simulink model "TestSolidStateTransformer"  (R2025b)
settings: Solver=VariableStepAuto  StartTime=0.0  StopTime=0.5  FixedStep=50e-6  RelTol=1e-3
model workspace (MAT data in the model file):
  sst : object (value not decoded)
  ups : sampleTime (value not decoded)
symbols that are objects in the model workspace (value not decoded): ups
undefined symbols (not defined in the file): DiscIntNeverNeededParam, ee_sli_rtmsupport, gcbh, Ts
libraries: fl_lib x23, nesl_utility x20, datacenter_lib x12, ee_lib x9, simulink x8, eeGeneralControl x6, eeTransforms x4, slpidlib x3, eeSinusoidalMeasurementV2 x2, simulink_extras x1
(part 2 of 2)

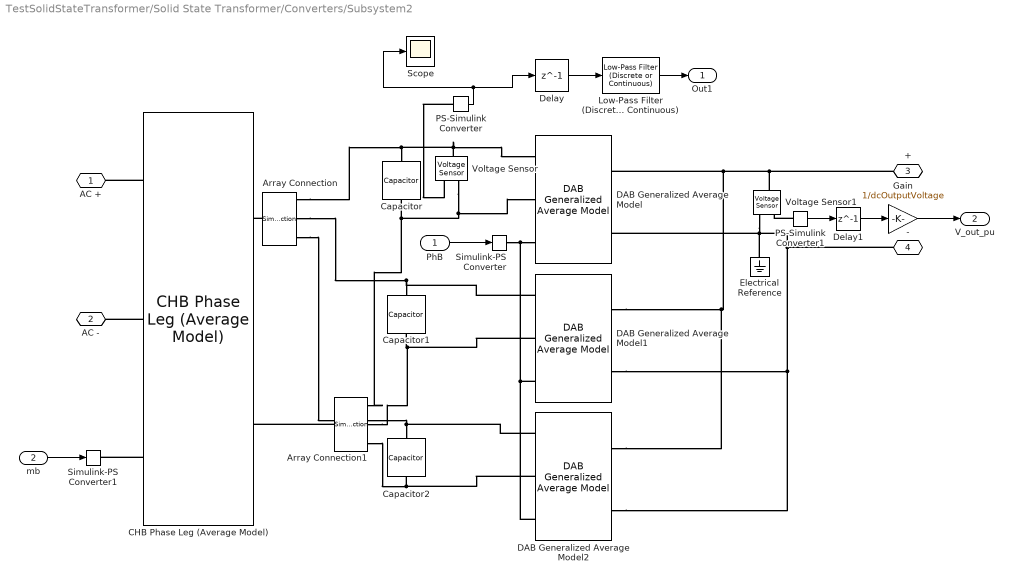
== system TestSolidStateTransformer/Solid State Transformer/Converters/Subsystem2 ==
  PhB : Inport
  mb : Inport  Port=2
  Array Connection : SimscapeArrayConnection  NumScalarElements=3
  Array Connection1 : SimscapeArrayConnection  NumScalarElements=3
  CHB Phase Leg (Average Model) : datacenter_lib/CHB Phase Leg (Average Model)  NumModules=3  OnResistance=1e-3 Ohm  InitialDCVoltage=4400 V  GridVoltage=13800 V  TotalDCVoltage=13200 V
      settings: InternalSimscapePortConfiguration="{\"Bottom\":[],\"Left\":[{\"id\":\"ACPositive\",\"label\":\"AC+\",\"type\":\"foundation.electrical.electrical\"},{\"id\":\"ACNegative\",\"label\":\"AC-\",\"type\":\"foundation.electrical.electrical\"},{\"id\":\"m\",\"label\":\"m\",\"type\":\"input\"}],\"Right\":[{\"id\":\"DCPositive\",\"label\":\"DC+\",\"type\":\"foundation.electrical.electrical\"},{\"id\":\"DCNegative\",\"label\":\"DC-\",\"type\":\"foundation.electrical.electrical\"}],\"Top\":[]}"
  Capacitor : fl_lib/Electrical/Electrical Elements/Capacitor  c=0.005 F  r=1e-6 Ohm  g=0 1/Ohm  i_specify=off  i_priority=None  i=0 A  i_nominal_specify=off  i_nominal_value=1  i_nominal_unit=A  v_specify=off  v_priority=None  v=0 V  v_nominal_specify=off  v_nominal_value=1  v_nominal_unit=V  vc_specify=on  vc_priority=None  vc=4400 V  vc_nominal_specify=off  vc_nominal_value=1  vc_nominal_unit=V
  Capacitor1 : fl_lib/Electrical/Electrical Elements/Capacitor  c=0.005 F  r=1e-6 Ohm  g=0 1/Ohm  i_specify=off  i_priority=None  i=0 A  i_nominal_specify=off  i_nominal_value=1  i_nominal_unit=A  v_specify=off  v_priority=None  v=0 V  v_nominal_specify=off  v_nominal_value=1  v_nominal_unit=V  vc_specify=on  vc_priority=None  vc=4400 V  vc_nominal_specify=off  vc_nominal_value=1  vc_nominal_unit=V
  Capacitor2 : fl_lib/Electrical/Electrical Elements/Capacitor  c=0.005 F  r=1e-6 Ohm  g=0 1/Ohm  i_specify=off  i_priority=None  i=0 A  i_nominal_specify=off  i_nominal_value=1  i_nominal_unit=A  v_specify=off  v_priority=None  v=0 V  v_nominal_specify=off  v_nominal_value=1  v_nominal_unit=V  vc_specify=on  vc_priority=None  vc=4400 V  vc_nominal_specify=off  vc_nominal_value=1  vc_nominal_unit=V
  DAB Generalized Average Model : datacenter_lib/DAB Generalized Average Model  N=5.5  L1=3.4e-05 H  L2=1.12e-06 H  Rt=0.005 Ohm  Co=0.001 F  fs=20000 Hz  vo0_init=800 V  it1R_init=0 A  it1I_init=0 A  include_esr=false  Rc=0.25 Ohm  i_in_specify=on  i_in_priority=None  i_in=0 A  i_in_nominal_specify=off  i_in_nominal_value=1  i_in_nominal_unit=A  i_out_specify=on  i_out_priority=None  i_out=0 A  i_out_nominal_specify=off  i_out_nominal_value=1  i_out_nominal_unit=A  v_in_specify=on  v_in_priority=None  v_in=0 V  v_in_nominal_specify=off  v_in_nominal_value=1  v_in_nominal_unit=V  v_out_specify=on  v_out_priority=None  v_out=0 V  v_out_nominal_specify=off  v_out_nominal_value=1  v_out_nominal_unit=V
      settings: InternalSimscapePortConfiguration="{\"Bottom\":[],\"Left\":[{\"id\":\"p_in\",\"label\":\"V+\",\"type\":\"foundation.electrical.electrical\"},{\"id\":\"n_in\",\"label\":\"V-\",\"type\":\"foundation.electrical.electrical\"},{\"id\":\"d\",\"label\":\"d\",\"type\":\"input\"}],\"Right\":[{\"id\":\"p_out\",\"label\":\"Vo+\",\"type\":\"foundation.electrical.electrical\"},{\"id\":\"n_out\",\"label\":\"Vo-\",\"type\":\"foundation.electrical.electrical\"}],\"Top\":[]}"
  DAB Generalized Average Model1 : datacenter_lib/DAB Generalized Average Model  N=5.5  L1=3.4e-05 H  L2=1.12e-06 H  Rt=0.005 Ohm  Co=0.001 F  fs=20000 Hz  vo0_init=800 V  it1R_init=0 A  it1I_init=0 A  include_esr=false  Rc=0.25 Ohm  i_in_specify=on  i_in_priority=None  i_in=0 A  i_in_nominal_specify=off  i_in_nominal_value=1  i_in_nominal_unit=A  i_out_specify=on  i_out_priority=None  i_out=0 A  i_out_nominal_specify=off  i_out_nominal_value=1  i_out_nominal_unit=A  v_in_specify=on  v_in_priority=None  v_in=0 V  v_in_nominal_specify=off  v_in_nominal_value=1  v_in_nominal_unit=V  v_out_specify=on  v_out_priority=None  v_out=0 V  v_out_nominal_specify=off  v_out_nominal_value=1  v_out_nominal_unit=V
      settings: InternalSimscapePortConfiguration="{\"Bottom\":[],\"Left\":[{\"id\":\"p_in\",\"label\":\"V+\",\"type\":\"foundation.electrical.electrical\"},{\"id\":\"n_in\",\"label\":\"V-\",\"type\":\"foundation.electrical.electrical\"},{\"id\":\"d\",\"label\":\"d\",\"type\":\"input\"}],\"Right\":[{\"id\":\"p_out\",\"label\":\"Vo+\",\"type\":\"foundation.electrical.electrical\"},{\"id\":\"n_out\",\"label\":\"Vo-\",\"type\":\"foundation.electrical.electrical\"}],\"Top\":[]}"
  DAB Generalized Average Model2 : datacenter_lib/DAB Generalized Average Model  N=5.5  L1=3.4e-05 H  L2=1.12e-06 H  Rt=0.005 Ohm  Co=0.001 F  fs=20000 Hz  vo0_init=800 V  it1R_init=0 A  it1I_init=0 A  include_esr=false  Rc=0.25 Ohm  i_in_specify=on  i_in_priority=None  i_in=0 A  i_in_nominal_specify=off  i_in_nominal_value=1  i_in_nominal_unit=A  i_out_specify=on  i_out_priority=None  i_out=0 A  i_out_nominal_specify=off  i_out_nominal_value=1  i_out_nominal_unit=A  v_in_specify=on  v_in_priority=None  v_in=0 V  v_in_nominal_specify=off  v_in_nominal_value=1  v_in_nominal_unit=V  v_out_specify=on  v_out_priority=None  v_out=0 V  v_out_nominal_specify=off  v_out_nominal_value=1  v_out_nominal_unit=V
      settings: InternalSimscapePortConfiguration="{\"Bottom\":[],\"Left\":[{\"id\":\"p_in\",\"label\":\"V+\",\"type\":\"foundation.electrical.electrical\"},{\"id\":\"n_in\",\"label\":\"V-\",\"type\":\"foundation.electrical.electrical\"},{\"id\":\"d\",\"label\":\"d\",\"type\":\"input\"}],\"Right\":[{\"id\":\"p_out\",\"label\":\"Vo+\",\"type\":\"foundation.electrical.electrical\"},{\"id\":\"n_out\",\"label\":\"Vo-\",\"type\":\"foundation.electrical.electrical\"}],\"Top\":[]}"
  Delay : Delay  DelayLength=1
  Delay1 : Delay  DelayLength=1  InitialCondition=1
  Electrical Reference : fl_lib/Electrical/Electrical Elements/Electrical Reference
  Gain : Gain  Gain=1/dcOutputVoltage
  Low-Pass Filter (Discrete or Continuous) : eeGeneralControl/Low-Pass Filter (Discrete or Continuous)  K=1  T=0.005  B=inf  A=-inf  init_option=Inherited from block input  x0=0  Ts=-1
  PS-Simulink Converter : nesl_utility/PS-Simulink Converter  PhysicalDomain=network_engine_domain  SubClassName=ps_output  LeftPortType=input  RightPortType=output  PseudoPeriodic=off  Frequencies=[]  VectorFormat=inherit  Unit=inherit  AffineConversion=off
  PS-Simulink Converter1 : nesl_utility/PS-Simulink Converter  PhysicalDomain=network_engine_domain  SubClassName=ps_output  LeftPortType=input  RightPortType=output  PseudoPeriodic=off  Frequencies=[]  VectorFormat=inherit  Unit=inherit  AffineConversion=off
  Scope : Scope
      settings: ActiveDisplayYMinimum=-1  ActiveDisplayYMaximum=1
  Simulink-PS Converter : nesl_utility/Simulink-PS Converter  PhysicalDomain=network_engine_domain  SubClassName=ps_input  LeftPortType=input  RightPortType=output  PseudoPeriodic=off  Frequencies=[]  NoiseDistribution=none  NoiseParameters=[]  Unit=1  AffineConversion=off  FilteringAndDerivatives=provide  SimscapeFilterOrder=1  InputFilterTimeConstant=0.001  UdotUserProvided=0
  Simulink-PS Converter1 : nesl_utility/Simulink-PS Converter  PhysicalDomain=network_engine_domain  SubClassName=ps_input  LeftPortType=input  RightPortType=output  PseudoPeriodic=off  Frequencies=[]  NoiseDistribution=none  NoiseParameters=[]  Unit=1  AffineConversion=off  FilteringAndDerivatives=provide  SimscapeFilterOrder=1  InputFilterTimeConstant=0.001  UdotUserProvided=0
  Voltage Sensor : fl_lib/Electrical/Electrical Sensors/Voltage Sensor
  Voltage Sensor1 : fl_lib/Electrical/Electrical Sensors/Voltage Sensor
  AC + : PMIOPort  Side=Left
  AC - : PMIOPort  Port=2  Side=Left
  + : PMIOPort  Port=3  Side=Right
  - : PMIOPort  Port=4  Side=Right
  Out1 : Outport
  V_out_pu : Outport  Port=2
  wires:
  mb/1 -> Simulink-PS Converter1/1
  Gain/1 -> V_out_pu/1
  PhB/1 -> Simulink-PS Converter/1
  Delay1/1 -> Gain/1
  PS-Simulink Converter1/1 -> Delay1/1
  Low-Pass Filter (Discrete or Continuous)/1 -> Out1/1
  Delay/1 -> Low-Pass Filter (Discrete or Continuous)/1
  PS-Simulink Converter/1 -> Scope/1, Delay/1
  connections:
  CHB Phase Leg (Average Model)/LConn3 -- Simulink-PS Converter1/RConn1
  Array Connection1/RConn1 -- CHB Phase Leg (Average Model)/RConn2
  Array Connection/RConn1 -- CHB Phase Leg (Average Model)/RConn1
  DAB Generalized Average Model/LConn3 -- DAB Generalized Average Model1/LConn3 -- DAB Generalized Average Model2/LConn3 -- Simulink-PS Converter/RConn1
  PS-Simulink Converter1/LConn1 -- Voltage Sensor1/RConn1
  DAB Generalized Average Model1/RConn2 -- DAB Generalized Average Model2/RConn2 -- DAB Generalized Average Model/RConn2 -- Voltage Sensor1/RConn2 -- Electrical Reference/LConn1 -- -/RConn1
  DAB Generalized Average Model/RConn1 -- DAB Generalized Average Model1/RConn1 -- DAB Generalized Average Model2/RConn1 -- Voltage Sensor1/LConn1 -- +/RConn1
  Capacitor/RConn1 -- DAB Generalized Average Model/LConn2 -- Voltage Sensor/RConn2 -- Array Connection1/LConn1
  CHB Phase Leg (Average Model)/LConn2 -- AC -/RConn1
  Array Connection/LConn3 -- DAB Generalized Average Model2/LConn1 -- Capacitor2/LConn1
  Array Connection1/LConn3 -- Capacitor2/RConn1 -- DAB Generalized Average Model2/LConn2
  CHB Phase Leg (Average Model)/LConn1 -- AC +/RConn1
  Array Connection/LConn1 -- DAB Generalized Average Model/LConn1 -- Voltage Sensor/LConn1 -- Capacitor/LConn1
  Array Connection1/LConn2 -- DAB Generalized Average Model1/LConn2 -- Capacitor1/RConn1
  Array Connection/LConn2 -- Capacitor1/LConn1 -- DAB Generalized Average Model1/LConn1
  PS-Simulink Converter/LConn1 -- Voltage Sensor/RConn1

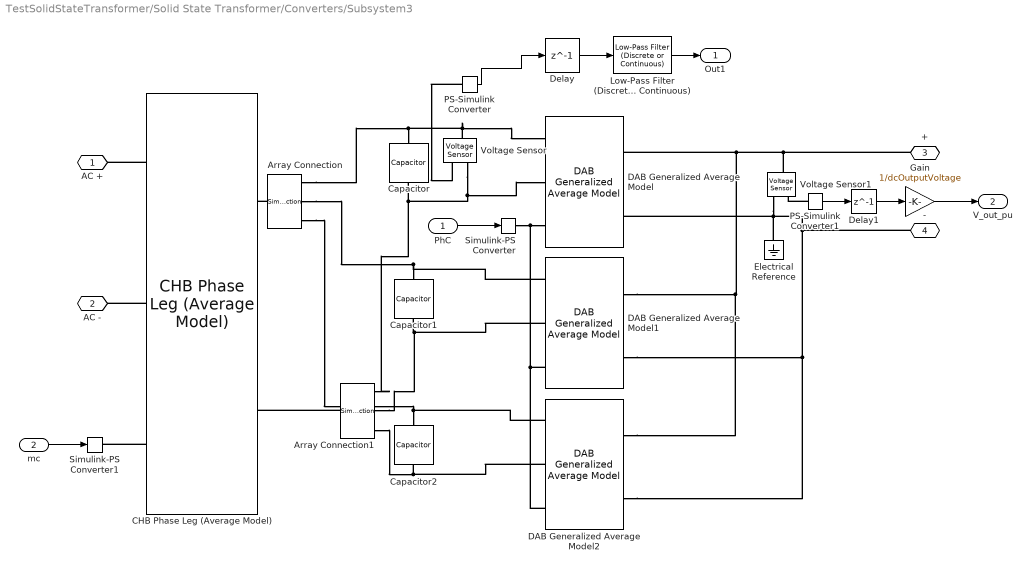
== system TestSolidStateTransformer/Solid State Transformer/Converters/Subsystem3 ==
  PhC : Inport
  mc : Inport  Port=2
  Array Connection : SimscapeArrayConnection  NumScalarElements=3
  Array Connection1 : SimscapeArrayConnection  NumScalarElements=3
  CHB Phase Leg (Average Model) : datacenter_lib/CHB Phase Leg (Average Model)  NumModules=3  OnResistance=1e-3 Ohm  InitialDCVoltage=4400 V  GridVoltage=13800 V  TotalDCVoltage=13200 V
      settings: InternalSimscapePortConfiguration="{\"Bottom\":[],\"Left\":[{\"id\":\"ACPositive\",\"label\":\"AC+\",\"type\":\"foundation.electrical.electrical\"},{\"id\":\"ACNegative\",\"label\":\"AC-\",\"type\":\"foundation.electrical.electrical\"},{\"id\":\"m\",\"label\":\"m\",\"type\":\"input\"}],\"Right\":[{\"id\":\"DCPositive\",\"label\":\"DC+\",\"type\":\"foundation.electrical.electrical\"},{\"id\":\"DCNegative\",\"label\":\"DC-\",\"type\":\"foundation.electrical.electrical\"}],\"Top\":[]}"
  Capacitor : fl_lib/Electrical/Electrical Elements/Capacitor  c=0.005 F  r=1e-6 Ohm  g=0 1/Ohm  i_specify=off  i_priority=None  i=0 A  i_nominal_specify=off  i_nominal_value=1  i_nominal_unit=A  v_specify=off  v_priority=None  v=0 V  v_nominal_specify=off  v_nominal_value=1  v_nominal_unit=V  vc_specify=on  vc_priority=None  vc=4400 V  vc_nominal_specify=off  vc_nominal_value=1  vc_nominal_unit=V
  Capacitor1 : fl_lib/Electrical/Electrical Elements/Capacitor  c=0.005 F  r=1e-6 Ohm  g=0 1/Ohm  i_specify=off  i_priority=None  i=0 A  i_nominal_specify=off  i_nominal_value=1  i_nominal_unit=A  v_specify=off  v_priority=None  v=0 V  v_nominal_specify=off  v_nominal_value=1  v_nominal_unit=V  vc_specify=on  vc_priority=None  vc=4400 V  vc_nominal_specify=off  vc_nominal_value=1  vc_nominal_unit=V
  Capacitor2 : fl_lib/Electrical/Electrical Elements/Capacitor  c=0.005 F  r=1e-6 Ohm  g=0 1/Ohm  i_specify=off  i_priority=None  i=0 A  i_nominal_specify=off  i_nominal_value=1  i_nominal_unit=A  v_specify=off  v_priority=None  v=0 V  v_nominal_specify=off  v_nominal_value=1  v_nominal_unit=V  vc_specify=on  vc_priority=None  vc=4400 V  vc_nominal_specify=off  vc_nominal_value=1  vc_nominal_unit=V
  DAB Generalized Average Model : datacenter_lib/DAB Generalized Average Model  N=5.5  L1=3.4e-05 H  L2=1.12e-06 H  Rt=0.005 Ohm  Co=0.001 F  fs=20000 Hz  vo0_init=800 V  it1R_init=0 A  it1I_init=0 A  include_esr=false  Rc=0.25 Ohm  i_in_specify=on  i_in_priority=None  i_in=0 A  i_in_nominal_specify=off  i_in_nominal_value=1  i_in_nominal_unit=A  i_out_specify=on  i_out_priority=None  i_out=0 A  i_out_nominal_specify=off  i_out_nominal_value=1  i_out_nominal_unit=A  v_in_specify=on  v_in_priority=None  v_in=0 V  v_in_nominal_specify=off  v_in_nominal_value=1  v_in_nominal_unit=V  v_out_specify=on  v_out_priority=None  v_out=0 V  v_out_nominal_specify=off  v_out_nominal_value=1  v_out_nominal_unit=V
      settings: InternalSimscapePortConfiguration="{\"Bottom\":[],\"Left\":[{\"id\":\"p_in\",\"label\":\"V+\",\"type\":\"foundation.electrical.electrical\"},{\"id\":\"n_in\",\"label\":\"V-\",\"type\":\"foundation.electrical.electrical\"},{\"id\":\"d\",\"label\":\"d\",\"type\":\"input\"}],\"Right\":[{\"id\":\"p_out\",\"label\":\"Vo+\",\"type\":\"foundation.electrical.electrical\"},{\"id\":\"n_out\",\"label\":\"Vo-\",\"type\":\"foundation.electrical.electrical\"}],\"Top\":[]}"
  DAB Generalized Average Model1 : datacenter_lib/DAB Generalized Average Model  N=5.5  L1=3.4e-05 H  L2=1.12e-06 H  Rt=0.005 Ohm  Co=0.001 F  fs=20000 Hz  vo0_init=800 V  it1R_init=0 A  it1I_init=0 A  include_esr=false  Rc=0.25 Ohm  i_in_specify=on  i_in_priority=None  i_in=0 A  i_in_nominal_specify=off  i_in_nominal_value=1  i_in_nominal_unit=A  i_out_specify=on  i_out_priority=None  i_out=0 A  i_out_nominal_specify=off  i_out_nominal_value=1  i_out_nominal_unit=A  v_in_specify=on  v_in_priority=None  v_in=0 V  v_in_nominal_specify=off  v_in_nominal_value=1  v_in_nominal_unit=V  v_out_specify=on  v_out_priority=None  v_out=0 V  v_out_nominal_specify=off  v_out_nominal_value=1  v_out_nominal_unit=V
      settings: InternalSimscapePortConfiguration="{\"Bottom\":[],\"Left\":[{\"id\":\"p_in\",\"label\":\"V+\",\"type\":\"foundation.electrical.electrical\"},{\"id\":\"n_in\",\"label\":\"V-\",\"type\":\"foundation.electrical.electrical\"},{\"id\":\"d\",\"label\":\"d\",\"type\":\"input\"}],\"Right\":[{\"id\":\"p_out\",\"label\":\"Vo+\",\"type\":\"foundation.electrical.electrical\"},{\"id\":\"n_out\",\"label\":\"Vo-\",\"type\":\"foundation.electrical.electrical\"}],\"Top\":[]}"
  DAB Generalized Average Model2 : datacenter_lib/DAB Generalized Average Model  N=5.5  L1=3.4e-05 H  L2=1.12e-06 H  Rt=0.005 Ohm  Co=0.001 F  fs=20000 Hz  vo0_init=800 V  it1R_init=0 A  it1I_init=0 A  include_esr=false  Rc=0.25 Ohm  i_in_specify=on  i_in_priority=None  i_in=0 A  i_in_nominal_specify=off  i_in_nominal_value=1  i_in_nominal_unit=A  i_out_specify=on  i_out_priority=None  i_out=0 A  i_out_nominal_specify=off  i_out_nominal_value=1  i_out_nominal_unit=A  v_in_specify=on  v_in_priority=None  v_in=0 V  v_in_nominal_specify=off  v_in_nominal_value=1  v_in_nominal_unit=V  v_out_specify=on  v_out_priority=None  v_out=0 V  v_out_nominal_specify=off  v_out_nominal_value=1  v_out_nominal_unit=V
      settings: InternalSimscapePortConfiguration="{\"Bottom\":[],\"Left\":[{\"id\":\"p_in\",\"label\":\"V+\",\"type\":\"foundation.electrical.electrical\"},{\"id\":\"n_in\",\"label\":\"V-\",\"type\":\"foundation.electrical.electrical\"},{\"id\":\"d\",\"label\":\"d\",\"type\":\"input\"}],\"Right\":[{\"id\":\"p_out\",\"label\":\"Vo+\",\"type\":\"foundation.electrical.electrical\"},{\"id\":\"n_out\",\"label\":\"Vo-\",\"type\":\"foundation.electrical.electrical\"}],\"Top\":[]}"
  Delay : Delay  DelayLength=1
  Delay1 : Delay  DelayLength=1  InitialCondition=1
  Electrical Reference : fl_lib/Electrical/Electrical Elements/Electrical Reference
  Gain : Gain  Gain=1/dcOutputVoltage
  Low-Pass Filter (Discrete or Continuous) : eeGeneralControl/Low-Pass Filter (Discrete or Continuous)  K=1  T=0.005  B=inf  A=-inf  init_option=Inherited from block input  x0=0  Ts=-1
  PS-Simulink Converter : nesl_utility/PS-Simulink Converter  PhysicalDomain=network_engine_domain  SubClassName=ps_output  LeftPortType=input  RightPortType=output  PseudoPeriodic=off  Frequencies=[]  VectorFormat=inherit  Unit=inherit  AffineConversion=off
  PS-Simulink Converter1 : nesl_utility/PS-Simulink Converter  PhysicalDomain=network_engine_domain  SubClassName=ps_output  LeftPortType=input  RightPortType=output  PseudoPeriodic=off  Frequencies=[]  VectorFormat=inherit  Unit=inherit  AffineConversion=off
  Simulink-PS Converter : nesl_utility/Simulink-PS Converter  PhysicalDomain=network_engine_domain  SubClassName=ps_input  LeftPortType=input  RightPortType=output  PseudoPeriodic=off  Frequencies=[]  NoiseDistribution=none  NoiseParameters=[]  Unit=1  AffineConversion=off  FilteringAndDerivatives=provide  SimscapeFilterOrder=1  InputFilterTimeConstant=0.001  UdotUserProvided=0
  Simulink-PS Converter1 : nesl_utility/Simulink-PS Converter  PhysicalDomain=network_engine_domain  SubClassName=ps_input  LeftPortType=input  RightPortType=output  PseudoPeriodic=off  Frequencies=[]  NoiseDistribution=none  NoiseParameters=[]  Unit=1  AffineConversion=off  FilteringAndDerivatives=provide  SimscapeFilterOrder=1  InputFilterTimeConstant=0.001  UdotUserProvided=0
  Voltage Sensor : fl_lib/Electrical/Electrical Sensors/Voltage Sensor
  Voltage Sensor1 : fl_lib/Electrical/Electrical Sensors/Voltage Sensor
  AC + : PMIOPort  Side=Left
  AC - : PMIOPort  Port=2  Side=Left
  + : PMIOPort  Port=3  Side=Right
  - : PMIOPort  Port=4  Side=Right
  Out1 : Outport
  V_out_pu : Outport  Port=2
  wires:
  mc/1 -> Simulink-PS Converter1/1
  Gain/1 -> V_out_pu/1
  PhC/1 -> Simulink-PS Converter/1
  Delay1/1 -> Gain/1
  PS-Simulink Converter1/1 -> Delay1/1
  Low-Pass Filter (Discrete or Continuous)/1 -> Out1/1
  Delay/1 -> Low-Pass Filter (Discrete or Continuous)/1
  PS-Simulink Converter/1 -> Delay/1
  connections:
  CHB Phase Leg (Average Model)/LConn3 -- Simulink-PS Converter1/RConn1
  Array Connection1/RConn1 -- CHB Phase Leg (Average Model)/RConn2
  Array Connection/RConn1 -- CHB Phase Leg (Average Model)/RConn1
  DAB Generalized Average Model/LConn3 -- DAB Generalized Average Model1/LConn3 -- DAB Generalized Average Model2/LConn3 -- Simulink-PS Converter/RConn1
  PS-Simulink Converter1/LConn1 -- Voltage Sensor1/RConn1
  DAB Generalized Average Model1/RConn2 -- DAB Generalized Average Model2/RConn2 -- DAB Generalized Average Model/RConn2 -- Voltage Sensor1/RConn2 -- Electrical Reference/LConn1 -- -/RConn1
  DAB Generalized Average Model/RConn1 -- DAB Generalized Average Model1/RConn1 -- DAB Generalized Average Model2/RConn1 -- Voltage Sensor1/LConn1 -- +/RConn1
  Capacitor/RConn1 -- DAB Generalized Average Model/LConn2 -- Voltage Sensor/RConn2 -- Array Connection1/LConn1
  CHB Phase Leg (Average Model)/LConn2 -- AC -/RConn1
  Array Connection/LConn3 -- DAB Generalized Average Model2/LConn1 -- Capacitor2/LConn1
  Array Connection1/LConn3 -- Capacitor2/RConn1 -- DAB Generalized Average Model2/LConn2
  CHB Phase Leg (Average Model)/LConn1 -- AC +/RConn1
  Array Connection/LConn1 -- DAB Generalized Average Model/LConn1 -- Voltage Sensor/LConn1 -- Capacitor/LConn1
  Array Connection1/LConn2 -- DAB Generalized Average Model1/LConn2 -- Capacitor1/RConn1
  Array Connection/LConn2 -- Capacitor1/LConn1 -- DAB Generalized Average Model1/LConn1
  PS-Simulink Converter/LConn1 -- Voltage Sensor/RConn1

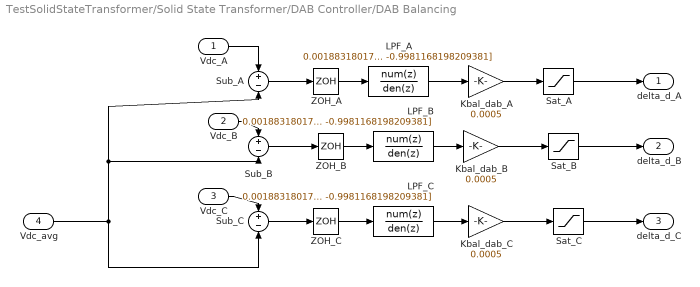
== system TestSolidStateTransformer/Solid State Transformer/DAB Controller/DAB Balancing ==
  Vdc_A : Inport
  Vdc_B : Inport  Port=2
  Vdc_C : Inport  Port=3
  Vdc_avg : Inport  Port=4
  Kbal_dab_A : Gain  Gain=0.0005
  Kbal_dab_B : Gain  Gain=0.0005
  Kbal_dab_C : Gain  Gain=0.0005
  LPF_A : DiscreteTransferFcn  Numerator=0.0018831801790618607  Denominator=[1, -0.9981168198209381]
  LPF_B : DiscreteTransferFcn  Numerator=0.0018831801790618607  Denominator=[1, -0.9981168198209381]
  LPF_C : DiscreteTransferFcn  Numerator=0.0018831801790618607  Denominator=[1, -0.9981168198209381]
  Sat_A : Saturate  UpperLimit=0.02  LowerLimit=-0.02
  Sat_B : Saturate  UpperLimit=0.02  LowerLimit=-0.02
  Sat_C : Saturate  UpperLimit=0.02  LowerLimit=-0.02
  Sub_A : Sum  Inputs=+-
  Sub_B : Sum  Inputs=+-
  Sub_C : Sum  Inputs=+-
  ZOH_A : ZeroOrderHold  SampleTime=2e-3
  ZOH_B : ZeroOrderHold  SampleTime=2e-3
  ZOH_C : ZeroOrderHold  SampleTime=2e-3
  delta_d_A : Outport
  delta_d_B : Outport  Port=2
  delta_d_C : Outport  Port=3
  wires:
  LPF_C/1 -> Kbal_dab_C/1
  ZOH_C/1 -> LPF_C/1
  LPF_B/1 -> Kbal_dab_B/1
  ZOH_B/1 -> LPF_B/1
  LPF_A/1 -> Kbal_dab_A/1
  ZOH_A/1 -> LPF_A/1
  Sat_C/1 -> delta_d_C/1
  Kbal_dab_C/1 -> Sat_C/1
  Sub_C/1 -> ZOH_C/1
  Sat_B/1 -> delta_d_B/1
  Kbal_dab_B/1 -> Sat_B/1
  Sub_B/1 -> ZOH_B/1
  Sat_A/1 -> delta_d_A/1
  Kbal_dab_A/1 -> Sat_A/1
  Sub_A/1 -> ZOH_A/1
  Vdc_C/1 -> Sub_C/1
  Vdc_B/1 -> Sub_B/1
  Vdc_avg/1 -> Sub_A/2, Sub_B/2, Sub_C/2
  Vdc_A/1 -> Sub_A/1

== system TestSolidStateTransformer/Solid State Transformer/Filter & AC measurements/Current ==
  Isabc : Inport
  Demux : Demux  Outputs=3
  Mux : Mux  Inputs=3
  Unit Delay : UnitDelay  SampleTime=-1
  Iabc : Outport
  wires:
  Demux/3 -> Mux/3
  Demux/2 -> Mux/2
  Demux/1 -> Mux/1
  Isabc/1 -> Unit Delay/1
  Unit Delay/1 -> Demux/1
  Mux/1 -> Iabc/1

== system TestSolidStateTransformer/Solid State Transformer/Filter & AC measurements/PLL ==
  Iabc : Inport
  V : Inport  Port=2
  Constant1 : Constant  Value=pi/2  SampleTime=Ts
  Data Type Conversion Inherited : simulink/Signal Attributes/Data Type Conversion Inherited  ConvertRealWorld=Real World Value  DoSatur=off
  Demux : Demux  Outputs=3
  Park Transform : eeTransforms/Park Transform  AxisAlignment=D-axis  PowerInvariant=off
  "Sinusoidal Measurement (PLL, Three-Phase)" : eeSinusoidalMeasurementV2/Sinusoidal Measurement (PLL, Three-Phase)  InputFilter=on  InputNormalization=off  Kp_LF=ups.AFE.kpPLL  Ki_LF=ups.AFE.kiPLL  F0=frequency  Theta0=0  Ts=Ts
  Sum : Sum  Inputs=|+-
  Terminator : Terminator
  Terminator2 : Terminator
  Id : Outport
  freq : Outport  Port=2
  mag : Outport  Port=3
  wires:
  "Sinusoidal Measurement (PLL, Three-Phase)"/3 -> mag/1
  Demux/2 -> Terminator2/1
  Iabc/1 -> Park Transform/1
  "Sinusoidal Measurement (PLL, Three-Phase)"/1 -> freq/1
  Demux/1 -> Id/1
  Sum/1 -> Park Transform/2
  Demux/3 -> Terminator/1
  Park Transform/1 -> Demux/1
  "Sinusoidal Measurement (PLL, Three-Phase)"/2 -> Data Type Conversion Inherited/1, Sum/1
  V/1 -> "Sinusoidal Measurement (PLL, Three-Phase)"/1
  Constant1/1 -> Data Type Conversion Inherited/2
  Data Type Conversion Inherited/1 -> Sum/2

== system TestSolidStateTransformer/Solid State Transformer/Filter & AC measurements/Voltage ==
  Vsabc : Inport
  Demux1 : Demux  Outputs=3
  Mux1 : Mux  Inputs=3
  Unit Delay : UnitDelay  SampleTime=-1
  Vabc : Outport
  wires:
  Demux1/3 -> Mux1/3
  Demux1/2 -> Mux1/2
  Demux1/1 -> Mux1/1
  Vsabc/1 -> Unit Delay/1
  Unit Delay/1 -> Demux1/1
  Mux1/1 -> Vabc/1

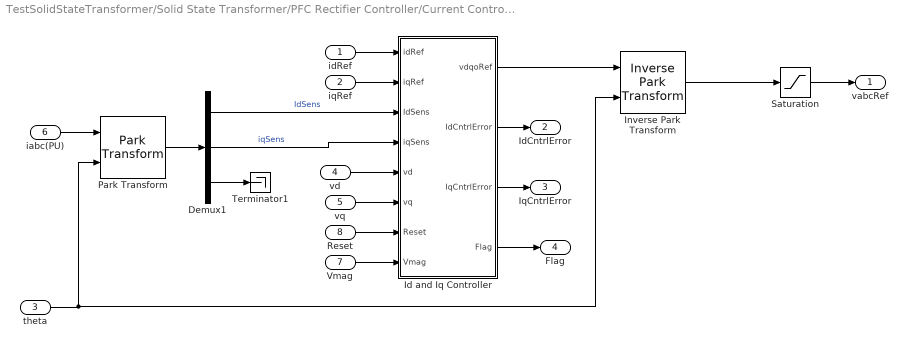
== system TestSolidStateTransformer/Solid State Transformer/PFC Rectifier Controller/Current Controller ==
  idRef : Inport
  iqRef : Inport  Port=2
  theta : Inport  Port=3
  vd : Inport  Port=4
  vq : Inport  Port=5
  iabc(PU) : Inport  Port=6
  Vmag : Inport  Port=7
  Reset : Inport  Port=8
  Demux1 : Demux  Outputs=3
  Id and Iq Controller : Subsystem
  Inverse Park Transform : eeTransforms/Inverse Park Transform  AxisAlignment=D-axis  PowerInvariant=off
  Park Transform : eeTransforms/Park Transform  AxisAlignment=D-axis  PowerInvariant=off
  Saturation : Saturate  UpperLimit=1.5  LowerLimit=-1.5
  Terminator1 : Terminator
  vabcRef : Outport
  IdCntrlError : Outport  Port=2
  IqCntrlError : Outport  Port=3
  Flag : Outport  Port=4
  wires:
  Id and Iq Controller/4(Flag) -> Flag/1
  Vmag/1 -> Id and Iq Controller/8(Vmag)
  Reset/1 -> Id and Iq Controller/7(Reset)
  Saturation/1 -> vabcRef/1
  Park Transform/1 -> Demux1/1
  Demux1/3 -> Terminator1/1
  theta/1 -> Inverse Park Transform/2, Park Transform/2
  iabc(PU)/1 -> Park Transform/1
  Inverse Park Transform/1 -> Saturation/1
  vd/1 -> Id and Iq Controller/5(vd)
  idRef/1 -> Id and Iq Controller/1(idRef)
  Demux1/1 -> Id and Iq Controller/3(IdSens)  "IdSens"
  iqRef/1 -> Id and Iq Controller/2(iqRef)
  Demux1/2 -> Id and Iq Controller/4(iqSens)  "iqSens"
  vq/1 -> Id and Iq Controller/6(vq)
  Id and Iq Controller/1(vdqoRef) -> Inverse Park Transform/1
  Id and Iq Controller/3(IqCntrlError) -> IqCntrlError/1
  Id and Iq Controller/2(IdCntrlError) -> IdCntrlError/1

== system TestSolidStateTransformer/Solid State Transformer/PFC Rectifier Controller/DC Voltage Controller and Current Reference ==
  qRef : Inport
  vPeak : Inport  Port=2
  vdcRef : Inport  Port=3
  VdcSens : Inport  Port=4
  Reset : Inport  Port=5
  Constant : Constant  SampleTime=Ts
  Data Type Conversion Inherited : simulink/Signal Attributes/Data Type Conversion Inherited  ConvertRealWorld=Real World Value  DoSatur=off
  Gain : Gain  Gain=-1
  Iq Reference : Subsystem
  Switch : Switch  Criteria=u2 > Threshold  SaturateOnIntegerOverflow=off  InputSameDT=off
  Voltage Controller : Subsystem
  idRef : Outport
  iqRef : Outport  Port=2
  wires:
  Reset/1 -> Voltage Controller/3(Reset)
  Switch/1 -> Iq Reference/1(V_mag)
  vPeak/1 -> Data Type Conversion Inherited/1, Switch/1, Switch/2
  Iq Reference/1(iq_ref) -> Gain/1
  VdcSens/1 -> Voltage Controller/2(Vdcmeas)
  vdcRef/1 -> Voltage Controller/1(Vdcref)
  Voltage Controller/1(Id) -> idRef/1
  qRef/1 -> Iq Reference/2(Q_ref)
  Gain/1 -> iqRef/1
  Data Type Conversion Inherited/1 -> Switch/3
  Constant/1 -> Data Type Conversion Inherited/2

== system TestSolidStateTransformer/Solid State Transformer/PFC Rectifier Controller/PLL ==
  V : Inport
  Constant1 : Constant  Value=pi/2  SampleTime=Ts
  Data Type Conversion Inherited : simulink/Signal Attributes/Data Type Conversion Inherited  ConvertRealWorld=Real World Value  DoSatur=off
  Demux : Demux  Outputs=3
  Filtered Derivative (Discrete or Continuous) : eeGeneralControl/Filtered Derivative (Discrete or Continuous)  K=1  T=0.005  B=inf  A=-inf  minRatio=10  init_option=Inherited from block input  x0=0  Ts=-1
      settings: LibrarySourceBlock=|
      | ee_sl_lib/General Control/Filtered Derivative
      | (Discrete or Continuous)
  Park Transform : eeTransforms/Park Transform  AxisAlignment=D-axis  PowerInvariant=off
  Scope : Scope  NumInputPorts=2
      settings: ActiveDisplayYMinimum=-0.12536761024201581  ActiveDisplayYMaximum=1.1283084921781426  DataLoggingVariableName=ScopeData20
  Scope1 : Scope
      settings: ActiveDisplayYMinimum=-1  ActiveDisplayYMaximum=1  DataLoggingVariableName=ScopeData21
  "Sinusoidal Measurement (PLL, Three-Phase)" : eeSinusoidalMeasurementV2/Sinusoidal Measurement (PLL, Three-Phase)  InputFilter=on  InputNormalization=off  Kp_LF=KpPLL  Ki_LF=KiPLL  F0=Freq  Theta0=0  Ts=Ts
  Sum : Sum  Inputs=|+-
  Terminator : Terminator
  Terminator1 : Terminator
  theta : Outport
  Vd : Outport  Port=2
  Vq : Outport  Port=3
  mag : Outport  Port=4
  wires:
  Filtered Derivative (Discrete or Continuous)/1 -> Scope1/1
  "Sinusoidal Measurement (PLL, Three-Phase)"/1 -> Terminator1/1
  Demux/1 -> Vd/1, Filtered Derivative (Discrete or Continuous)/1, Scope/2
  Demux/2 -> Vq/1
  Sum/1 -> theta/1, Park Transform/2
  "Sinusoidal Measurement (PLL, Three-Phase)"/3 -> mag/1, Scope/1
  Demux/3 -> Terminator/1
  Park Transform/1 -> Demux/1
  "Sinusoidal Measurement (PLL, Three-Phase)"/2 -> Data Type Conversion Inherited/1, Sum/1
  V/1 -> "Sinusoidal Measurement (PLL, Three-Phase)"/1, Park Transform/1
  Constant1/1 -> Data Type Conversion Inherited/2
  Data Type Conversion Inherited/1 -> Sum/2

== system TestSolidStateTransformer/Solid State Transformer/PFC Rectifier Controller/Reset Controller ==
  u : Inport
  AND : Logic  IconShape=distinctive  AllPortsSameDT=off  OutDataTypeStr=boolean
  AND1 : Logic  IconShape=distinctive  AllPortsSameDT=off  OutDataTypeStr=boolean
  Compare To Constant : simulink/Logic and Bit Operations/Compare To Constant  relop=<=  const=0.5  OutDataTypeStr=boolean
  Compare To Constant1 : simulink/Logic and Bit Operations/Compare To Constant  relop=>  const=0.5  OutDataTypeStr=boolean
  Compare To Constant2 : simulink/Logic and Bit Operations/Compare To Constant  relop=>  const=0.05  OutDataTypeStr=boolean
  Data Type Conversion : DataTypeConversion  SaturateOnIntegerOverflow=off  RndMeth=Floor
  Data Type Conversion1 : DataTypeConversion  OutDataTypeStr=double  SaturateOnIntegerOverflow=off  RndMeth=Floor
  Delay : Delay  DelayLength=1
  Discrete-Time Integrator : DiscreteIntegrator  IntegratorMethod=Integration: Backward Euler  ExternalReset=falling  SampleTime=ups.sampleTime  LimitOutput=on  UpperSaturationLimit=0.6  LowerSaturationLimit=0  ICPrevOutput=DiscIntNeverNeededParam  ICPrevScaledInput=DiscIntNeverNeededParam
  NOT : Logic  Operator=NOT  IconShape=distinctive  AllPortsSameDT=off  OutDataTypeStr=boolean
  S-R Flip-Flop : simulink_extras/Flip Flops/S-R Flip-Flop  initial_condition=0
  Scope2 : Scope
      settings: ActiveDisplayYMinimum=-0.12499999999999997  ActiveDisplayYMaximum=1.125  DataLoggingVariableName=ScopeData8
  Out1 : Outport
  wires:
  NOT/1 -> Out1/1
  Data Type Conversion/1 -> S-R Flip-Flop/2
  Compare To Constant2/1 -> AND1/2
  AND/1 -> S-R Flip-Flop/1, Scope2/1
  AND1/1 -> Data Type Conversion/1
  S-R Flip-Flop/1 -> NOT/1
  Delay/1 -> Compare To Constant/1
  Data Type Conversion1/1 -> AND1/1, Discrete-Time Integrator/1, Discrete-Time Integrator/2
  Discrete-Time Integrator/1 -> Compare To Constant2/1
  Compare To Constant/1 -> AND/1
  Compare To Constant1/1 -> AND/2, Data Type Conversion1/1
  u/1 -> Delay/1, Compare To Constant1/1

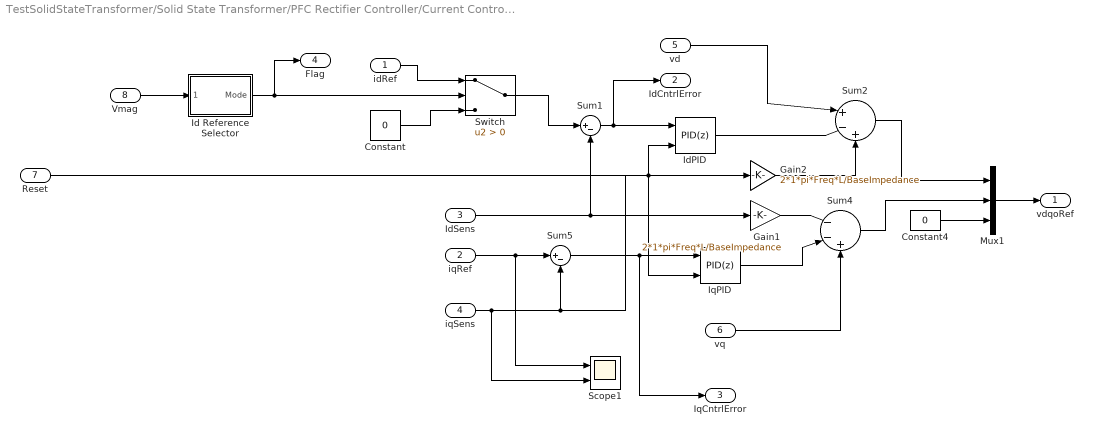
== system TestSolidStateTransformer/Solid State Transformer/PFC Rectifier Controller/Current Controller/Id and Iq Controller ==
  idRef : Inport
  iqRef : Inport  Port=2
  IdSens : Inport  Port=3
  iqSens : Inport  Port=4
  vd : Inport  Port=5
  vq : Inport  Port=6
  Reset : Inport  Port=7
  Vmag : Inport  Port=8
  Constant : Constant  Value=0
  Constant4 : Constant  Value=0
  Gain1 : Gain  Gain=2*1*pi*Freq*L/BaseImpedance
  Gain2 : Gain  Gain=2*1*pi*Freq*L/BaseImpedance
  Id Reference Selector : Subsystem
  IdPID : slpidlib/PID Controller  Controller=PID  Form=Parallel  TimeDomain=Discrete-time  UseExternalTs=off  SampleTime=Ts  IntegratorMethod=Forward Euler  FilterMethod=Forward Euler  ControllerParametersSource=internal  P=KpdCurrent  I=KidCurrent  UseKiTs=off  D=KddCurrent  UseExternalDerivativeSource=off  N=NdCurrent  UseFilter=on  TunerSelectOption=Transfer Function Based (PID Tuner App)  InitialConditionSource=internal  InitialConditionForIntegrator=0  InitialConditionForFilter=0  DifferentiatorICPrevScaledInput=0  ExternalReset=falling  TrackingMode=off  Kt=1  LimitOutput=on  SatLimitsSource=internal  UpperSaturationLimit=IdControlUpperLimit  LowerSaturationLimit=IdControlLowerLimit  LinearizeAsGain=on  AntiWindupMode=clamping  Kb=1  LimitIntegrator=on  UpperIntegratorSaturationLimit=IdControlUpperLimit  LowerIntegratorSaturationLimit=IdControlLowerLimit  POutMin=[]  POutMax=[]  IOutMin=[]  IOutMax=[]  DOutMin=[]  DOutMax=[]  NOutMin=[]  NOutMax=[]  SumOutMin=[]  SumOutMax=[]  SaturationOutMin=[]  SaturationOutMax=[]  PParamMin=[]  PParamMax=[]  IParamMin=[]  IParamMax=[]  DParamMin=[]  DParamMax=[]  NParamMin=[]  NParamMax=[]  KbParamMin=[]  KbParamMax=[]  KtParamMin=[]  KtParamMax=[]  KbOutMin=[]  KbOutMax=[]  KtOutMin=[]  KtOutMax=[]  IntegratorOutMin=[]  IntegratorOutMax=[]  FilterOutMin=[]  FilterOutMax=[]  SumI1OutMin=[]  SumI1OutMax=[]  SumI2OutMin=[]  SumI2OutMax=[]  SumI3OutMin=[]  SumI3OutMax=[]  SumI4OutMin=[]  SumI4OutMax=[]  SumDOutMin=[]  SumDOutMax=[]  DifferentiatorOutMin=[]  DifferentiatorOutMax=[]  FilterDiffOutCoefMin=[]  FilterDiffOutCoefMax=[]  ReciprocalOutMin=[]  ReciprocalOutMax=[]  SumDenOutMin=[]  SumDenOutMax=[]  SumNumOutMin=[]  SumNumOutMax=[]  DivideOutMin=[]  DivideOutMax=[]  UdiffTsProdOutMin=[]  UdiffTsProdOutMax=[]  NTsProdOutMin=[]  NTsProdOutMax=[]  UintegralTsProdOutMin=[]  UintegralTsProdOutMax=[]  UngainTsProdOutMin=[]  UngainTsProdOutMax=[]  ClampingZeroOutDataTypeStr=Inherit: Inherit via back propagation  ClampingZeroOutMin=[]  ClampingZeroOutMax=[]  FilterDenConstantOutDataTypeStr=Inherit: Inherit via back propagation  FilterDenConstantOutMin=[]  FilterDenConstantOutMax=[]  PCopyOutDataTypeStr=Inherit: Inherit via back propagation  PCopyOutMin=[]  PCopyOutMax=[]  NCopyOutDataTypeStr=Inherit: Inherit via back propagation  NCopyOutMin=[]  NCopyOutMax=[]  IntegratorContinuousStateAttributes=''  IntegratorStateMustResolveToSignalObject=off  IntegratorRTWStateStorageClass=Auto  FilterContinuousStateAttributes=''  FilterStateMustResolveToSignalObject=off  FilterRTWStateStorageClass=Auto  ParallelPVariant=InternalParameters  IdealPVariant=Disabled  IVariant=InternalParameters  DVariant=InternalParameters  IntegratorVariant=Discrete  SatVariant=Enabled  AWVariant=DiscClampingParallel  PCopyVariant=Disabled  TRVariant=Disabled  FdbkBlocksVariant=Forward  IdealPFdbkVariant=Disabled  SatFdbkVariant=Disabled  DerivativeFilterVariant=ForwardEulerFilter  NVariant=InternalParameters  NCopyVariant=Disabled  FilterICVariant=InternalICsFilter  IntegratorICVariant=InternalICs  ExternalResetVariant=ExternalReset  TRSumVariant=Passthrough  SumFdbkVariant=Disabled  SumVariant=Sum_PID  TsampFilterVariant=InternalTs  TsampNgainVariant=Passthrough  TsampIntegralVariant=Disabled_SignalSpec  ExternalSaturationOutDataTypeStr=Inherit: Same as second input  DerivativeSourceVariant=ErrorSignal  PreIntVariant=InternalPreInt
  IqPID : slpidlib/PID Controller  Controller=PID  Form=Parallel  TimeDomain=Discrete-time  UseExternalTs=off  SampleTime=Ts  IntegratorMethod=Forward Euler  FilterMethod=Forward Euler  ControllerParametersSource=internal  P=KpqCurrent  I=KiqCurrent  UseKiTs=off  D=KdqCurrent  UseExternalDerivativeSource=off  N=NdCurrent  UseFilter=on  TunerSelectOption=Transfer Function Based (PID Tuner App)  InitialConditionSource=internal  InitialConditionForIntegrator=0  InitialConditionForFilter=0  DifferentiatorICPrevScaledInput=0  ExternalReset=falling  TrackingMode=off  Kt=1  LimitOutput=on  SatLimitsSource=internal  UpperSaturationLimit=IqControlUpperLimit  LowerSaturationLimit=IqControlLowerLimit  LinearizeAsGain=on  AntiWindupMode=clamping  Kb=1  LimitIntegrator=on  UpperIntegratorSaturationLimit=IqControlUpperLimit  LowerIntegratorSaturationLimit=IqControlLowerLimit  POutMin=[]  POutMax=[]  IOutMin=[]  IOutMax=[]  DOutMin=[]  DOutMax=[]  NOutMin=[]  NOutMax=[]  SumOutMin=[]  SumOutMax=[]  SaturationOutMin=[]  SaturationOutMax=[]  PParamMin=[]  PParamMax=[]  IParamMin=[]  IParamMax=[]  DParamMin=[]  DParamMax=[]  NParamMin=[]  NParamMax=[]  KbParamMin=[]  KbParamMax=[]  KtParamMin=[]  KtParamMax=[]  KbOutMin=[]  KbOutMax=[]  KtOutMin=[]  KtOutMax=[]  IntegratorOutMin=[]  IntegratorOutMax=[]  FilterOutMin=[]  FilterOutMax=[]  SumI1OutMin=[]  SumI1OutMax=[]  SumI2OutMin=[]  SumI2OutMax=[]  SumI3OutMin=[]  SumI3OutMax=[]  SumI4OutMin=[]  SumI4OutMax=[]  SumDOutMin=[]  SumDOutMax=[]  DifferentiatorOutMin=[]  DifferentiatorOutMax=[]  FilterDiffOutCoefMin=[]  FilterDiffOutCoefMax=[]  ReciprocalOutMin=[]  ReciprocalOutMax=[]  SumDenOutMin=[]  SumDenOutMax=[]  SumNumOutMin=[]  SumNumOutMax=[]  DivideOutMin=[]  DivideOutMax=[]  UdiffTsProdOutMin=[]  UdiffTsProdOutMax=[]  NTsProdOutMin=[]  NTsProdOutMax=[]  UintegralTsProdOutMin=[]  UintegralTsProdOutMax=[]  UngainTsProdOutMin=[]  UngainTsProdOutMax=[]  ClampingZeroOutDataTypeStr=Inherit: Inherit via back propagation  ClampingZeroOutMin=[]  ClampingZeroOutMax=[]  FilterDenConstantOutDataTypeStr=Inherit: Inherit via back propagation  FilterDenConstantOutMin=[]  FilterDenConstantOutMax=[]  PCopyOutDataTypeStr=Inherit: Inherit via back propagation  PCopyOutMin=[]  PCopyOutMax=[]  NCopyOutDataTypeStr=Inherit: Inherit via back propagation  NCopyOutMin=[]  NCopyOutMax=[]  IntegratorContinuousStateAttributes=''  IntegratorStateMustResolveToSignalObject=off  IntegratorRTWStateStorageClass=Auto  FilterContinuousStateAttributes=''  FilterStateMustResolveToSignalObject=off  FilterRTWStateStorageClass=Auto  ParallelPVariant=InternalParameters  IdealPVariant=Disabled  IVariant=InternalParameters  DVariant=InternalParameters  IntegratorVariant=Discrete  SatVariant=Enabled  AWVariant=DiscClampingParallel  PCopyVariant=Disabled  TRVariant=Disabled  FdbkBlocksVariant=Forward  IdealPFdbkVariant=Disabled  SatFdbkVariant=Disabled  DerivativeFilterVariant=ForwardEulerFilter  NVariant=InternalParameters  NCopyVariant=Disabled  FilterICVariant=InternalICsFilter  IntegratorICVariant=InternalICs  ExternalResetVariant=ExternalReset  TRSumVariant=Passthrough  SumFdbkVariant=Disabled  SumVariant=Sum_PID  TsampFilterVariant=InternalTs  TsampNgainVariant=Passthrough  TsampIntegralVariant=Disabled_SignalSpec  ExternalSaturationOutDataTypeStr=Inherit: Same as second input  DerivativeSourceVariant=ErrorSignal  PreIntVariant=InternalPreInt
  Mux1 : Mux  Inputs=3
  Scope1 : Scope  NumInputPorts=2
      settings: ActiveDisplayYMinimum=-1  ActiveDisplayYMaximum=1  DataLoggingVariableName=ScopeData10
  Sum1 : Sum  Inputs=|+-
  Sum2 : Sum  Inputs=|+-+
  Sum4 : Sum  Inputs=|--+
  Sum5 : Sum  Inputs=|+-
  Switch : Switch  Criteria=u2 > Threshold  SaturateOnIntegerOverflow=off  InputSameDT=off
  vdqoRef : Outport
  IdCntrlError : Outport  Port=2
  IqCntrlError : Outport  Port=3
  Flag : Outport  Port=4
  wires:
  Switch/1 -> Sum1/1
  Vmag/1 -> Id Reference Selector/1(Vmag)
  Id Reference Selector/1(Mode) -> Switch/2, Flag/1
  iqRef/1 -> Sum5/1, Scope1/1
  Constant/1 -> Switch/3
  Constant4/1 -> Mux1/3
  Reset/1 -> IqPID/2, IdPID/2
  Sum5/1 -> IqCntrlError/1, IqPID/1
  Sum4/1 -> Mux1/2
  Sum2/1 -> Mux1/1
  iqSens/1 -> Sum5/2, Gain2/1, Scope1/2
  vq/1 -> Sum4/3
  Gain1/1 -> Sum4/1
  Gain2/1 -> Sum2/3
  IdPID/1 -> Sum2/2
  vd/1 -> Sum2/1
  Sum1/1 -> IdCntrlError/1, IdPID/1
  IdSens/1 -> Sum1/2, Gain1/1
  IqPID/1 -> Sum4/2
  idRef/1 -> Switch/1
  Mux1/1 -> vdqoRef/1

== system TestSolidStateTransformer/Solid State Transformer/PFC Rectifier Controller/DC Voltage Controller and Current Reference/Iq Reference ==
  V_mag : Inport
  Q_ref : Inport  Port=2
  Divide2 : Product  Inputs=*/
  iq_ref : Outport
  wires:
  Divide2/1 -> iq_ref/1
  Q_ref/1 -> Divide2/1
  V_mag/1 -> Divide2/2

== system TestSolidStateTransformer/Solid State Transformer/PFC Rectifier Controller/DC Voltage Controller and Current Reference/Voltage Controller ==
  Vdcref : Inport
  Vdcmeas : Inport  Port=2
  Reset : Inport  Port=3
  Gain : Gain  Gain=1/BaseVdc
  Saturation : Saturate  UpperLimit=1.0  LowerLimit=0
  Scope : Scope  NumInputPorts=2
      settings: ActiveDisplayYMinimum=-1  ActiveDisplayYMaximum=1  DataLoggingVariableName=ScopeData14
  Sum : Sum  Inputs=|+-
  Voltage control : Subsystem
  Id : Outport
  wires:
  Saturation/1 -> Id/1
  Reset/1 -> Voltage control/2(Reset)
  Voltage control/1(u) -> Saturation/1
  Vdcref/1 -> Sum/1, Scope/1
  Vdcmeas/1 -> Sum/2, Scope/2
  Gain/1 -> Voltage control/1(e)
  Sum/1 -> Gain/1

== system TestSolidStateTransformer/Solid State Transformer/PFC Rectifier Controller/Current Controller/Id and Iq Controller/Id Reference Selector ==
  Vmag : Inport
  AND1 : Logic  IconShape=distinctive  AllPortsSameDT=off  OutDataTypeStr=boolean
  Bias : Bias  Bias=0.01  SaturateOnIntegerOverflow=off
  Compare To Constant : simulink/Logic and Bit Operations/Compare To Constant  relop=>  const=0.5  OutDataTypeStr=boolean
  Compare To Constant2 : simulink/Logic and Bit Operations/Compare To Constant  relop=>  const=0.05  OutDataTypeStr=boolean
  Data Type Conversion : DataTypeConversion  SaturateOnIntegerOverflow=off  RndMeth=Floor
  Data Type Conversion1 : DataTypeConversion  OutDataTypeStr=double  SaturateOnIntegerOverflow=off  RndMeth=Floor
  Discrete-Time Integrator : DiscreteIntegrator  IntegratorMethod=Integration: Backward Euler  ExternalReset=falling  SampleTime=ups.sampleTime  LimitOutput=on  UpperSaturationLimit=0.6  LowerSaturationLimit=0  ICPrevOutput=DiscIntNeverNeededParam  ICPrevScaledInput=DiscIntNeverNeededParam
  Mode : Outport
  wires:
  Bias/1 -> Compare To Constant/1
  Vmag/1 -> Bias/1
  Compare To Constant/1 -> Data Type Conversion1/1
  AND1/1 -> Data Type Conversion/1
  Compare To Constant2/1 -> AND1/2
  Discrete-Time Integrator/1 -> Compare To Constant2/1
  Data Type Conversion1/1 -> AND1/1, Discrete-Time Integrator/1, Discrete-Time Integrator/2
  Data Type Conversion/1 -> Mode/1

== system TestSolidStateTransformer/Solid State Transformer/PFC Rectifier Controller/DC Voltage Controller and Current Reference/Voltage Controller/Voltage control ==
  e : Inport
  Reset : Inport  Port=2
  Discrete-Time Integrator : DiscreteIntegrator  IntegratorMethod=Integration: Backward Euler  ExternalReset=falling  SampleTime=ups.sampleTime  LimitOutput=on  UpperSaturationLimit=1  LowerSaturationLimit=0  ICPrevOutput=DiscIntNeverNeededParam  ICPrevScaledInput=DiscIntNeverNeededParam
  Ki : Gain  Gain=KiVoltage
  Kp : Gain  Gain=KpVoltage
  Sum7 : Sum  Inputs=|++
  u : Outport  VectorParamsAs1DForOutWhenUnconnected=off
  wires:
  Reset/1 -> Discrete-Time Integrator/2
  Discrete-Time Integrator/1 -> Sum7/2
  Kp/1 -> Sum7/1
  Sum7/1 -> u/1
  Ki/1 -> Discrete-Time Integrator/1
  e/1 -> Kp/1, Ki/1
